simulink model "PhaseII_opalrt_NoProtection"  (Simulink 8.8)
settings: Solver=ode3  StartTime=0.0  StopTime=inf  FixedStep=Ts  RelTol=1e-5  EnableMultiTasking=on
PostLoadFcn:
  | %BESS ctrl
  | Kpf=0.005*3*12;
  | Kif=5*6;
  | 
  | Kpf1=0.005*3*12;
  | Kif1=5*6;
  | Kp_v=0.016*15*35;
  | Ki_v=12*25;
  | 
  | Kp_v1=0.016*15*35;
  | Ki_v1=12*25;
  | 
  | Vabc_B=12.47e3;
  | Vdc_ref=Vabc_B*2;
  | Kpwm=sqrt(2)*Vabc_B/Vdc_ref;
  | ZB=Vabc_B^2/1e6;
  | R=0.005*ZB;
  | Ibasefull=673/2*sqrt(2);
  | 
  | 
  | Ts_Control=1e-4;
  | ts=0.05;
  | delay=0.2;
  | offset=10e3;
  | t_plan=60;
  | t_monitor=.2;
  | t_mon=t_monitor;
  | scalingfactor=1;
  | x=0.5;
  | n=6;
  | %t_plan=1/15;
  | %t_monitor=10/900;
  | %t_mon=10/900;
  | 
  | %t_plan=1/5;
  | %t_monitor=10/300;
  | %t_mon=10/300;
  | %scalingfactor=1/300;
  | 
  | f0=60;
  | 
  | Pabc_B=1e6;
  | Iabc_B=Pabc_B*sqrt(2/3)/Vabc_B;  % pk value
  | Imax_1=2.5;
  | Ptrans_B=Pabc_B*200;
  | 
  | Vdc_ref=Vabc_B*2;
  | 
  | ZB=Vabc_B^2/Pabc_B;
  | L=0.1*ZB/2/pi/60;
  | R=0.1*ZB;
  | C=1/(4*pi^2*(2e3)^2*L);
  | 
  | LL=0.005*ZB/2/pi/60;
  | RR=0.005*ZB;
  | 
  | RC=0.02;
  | 
  | %%% Initial SOC %%%%
  | SOC_ini_BESS1=0.5;
  | ... (+223 lines)
InitFcn:
  | %BESS ctrl
  | Kpf=0.005*3*12;
  | Kif=5*6;
  | 
  | Kpf1=0.005*3*12;
  | Kif1=5*6;
  | Kp_v=0.016*15*35;
  | Ki_v=12*25;
  | 
  | Kp_v1=0.016*15*35;
  | Ki_v1=12*25;
  | 
  | Vabc_B=12.47e3;
  | Vdc_ref=Vabc_B*2;
  | Kpwm=sqrt(2)*Vabc_B/Vdc_ref;
  | ZB=Vabc_B^2/1e6;
  | R=0.005*ZB;
  | Ibasefull=673/2*sqrt(2);
  | 
  | 
  | Ts_Control=1e-4;
  | ts=0.05;
  | delay=0.2;
  | offset=10e3;
  | t_plan=60;
  | t_monitor=.2;
  | t_mon=t_monitor;
  | scalingfactor=1;
  | x=0.5;
  | n=6;
  | %t_plan=1/15;
  | %t_monitor=10/900;
  | %t_mon=10/900;
  | 
  | %t_plan=1/5;
  | %t_monitor=10/300;
  | %t_mon=10/300;
  | %scalingfactor=1/300;
  | 
  | f0=60;
  | 
  | Pabc_B=1e6;
  | Iabc_B=Pabc_B*sqrt(2/3)/Vabc_B;  % pk value
  | Imax_1=2.5;
  | Ptrans_B=Pabc_B*200;
  | 
  | Vdc_ref=Vabc_B*2;
  | 
  | ZB=Vabc_B^2/Pabc_B;
  | L=0.1*ZB/2/pi/60;
  | R=0.1*ZB;
  | C=1/(4*pi^2*(2e3)^2*L);
  | 
  | LL=0.005*ZB/2/pi/60;
  | RR=0.005*ZB;
  | 
  | RC=0.02;
  | 
  | %%% Initial SOC %%%%
  | SOC_ini_BESS1=0.5;
  | ... (+223 lines)
undefined symbols (not defined in the file): D1, Delta, DiscIntNeverNeededParam, Left, PG2ref, type, V
libraries: powerlib x220, powerlib_meascontrol x82, dspstat3 x54, dsparch4 x43, dspswit3 x24, simulink x19, simulink_extras x12, powerlib_extras x11, ssn_lib x7, artemis x6, rtlab x5, rtio_generic_dnp3 x5
(part 5 of 9)

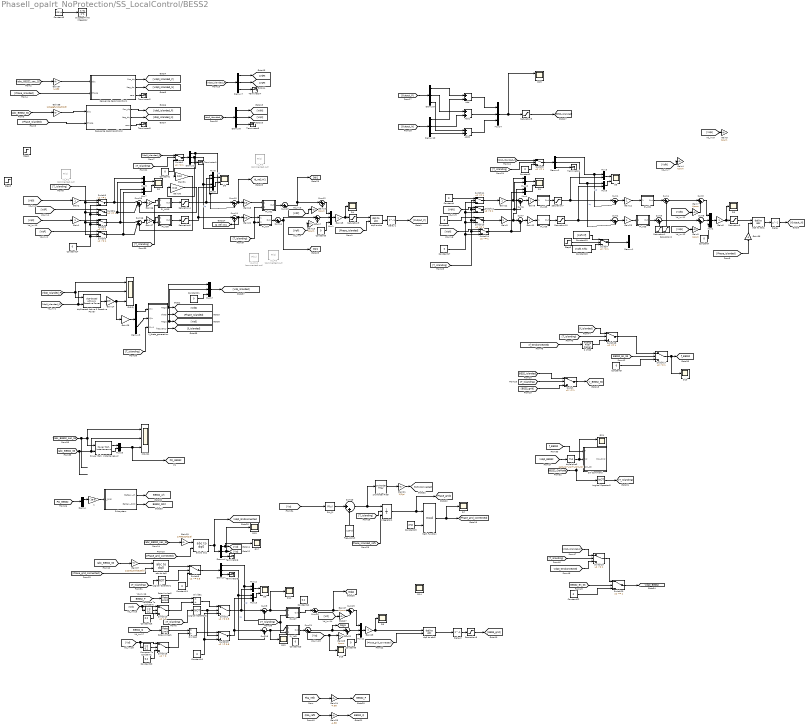
== system PhaseII_opalrt_NoProtection/SS_LocalControl/BESS2 ==
  "     1" : Gain  Gain=-1e-6
  2 kHz5 : dsparch4/Analog Filter Design  method=Butterworth  filttype=Lowpass  N=2  Wlo=2*pi*1  Whi=80  Rp=2  Rs=40
  2nd-Order Filter : powerlib_extras/Control  Blocks/2nd-Order Filter  FilterType=Lowpass  Fo=25  Zeta=0.707  Initialize=on  Vac_Init=[0 0 60]  Vdc_Init=377  PlotResponse=off  param1=[1 1000 0.5]
  Add : Sum
  Add1 : Sum
  Add2 : Sum
  Compare To Constant : simulink/Logic and Bit Operations/Compare To Constant  relop=>=  const=0.2  OutDataTypeStr=boolean
  Compare To Constant1 : simulink/Logic and Bit Operations/Compare To Constant  relop=>=  const=0.2  OutDataTypeStr=boolean
  Constant{1..2,4..11,13..14,17,21..22} (15 alike) : Constant  Value=0  SampleTime=-1
  Constant12 : Constant  Value=0.1  SampleTime=-1
  Constant15 : Constant  Value=2*pi
  Constant16 : Constant  Value=0.2  SampleTime=-1
  Constant18 : Constant  Value=[Kpf1 Kif1]  SampleTime=-1
  Constant19 : Constant  Value=[Kpf Kif]  SampleTime=-1
  Constant20 : Constant  Value=0.2  SampleTime=-1
  Constant3 : Constant  Value=120*pi
  D{1..2,5..6,9,15} (6 alike) : Scope  NumInputPorts=2
  D{3..4,7..8,10..14,16..17} (11 alike) : Scope
  D21 : Scope  NumInputPorts=3
  Delay : Delay  DelayLength=1  InitialCondition=0
  Delay1 : Delay  DelayLength=1  InitialCondition=0
  Delay2 : Delay  DelayLength=1  InitialCondition=0
  Demux : Demux  Outputs=2
  Demux1 : Demux  Outputs=2
  Demux{2,4..10} (8 alike) : Demux  Outputs=3
  Demux3 : Demux  Outputs=2
  Discrete-Time Integrator : DiscreteIntegrator  SampleTime=-1  ICPrevOutput=DiscIntNeverNeededParam  ICPrevScaledInput=DiscIntNeverNeededParam
  Divide1 : Product  Inputs=*/
  Divide2 : Product  Inputs=*/
  Freq_Const : Constant  Value=120*pi
  Gain{1..3,6,8,11..12,15,22..23,29} (11 alike) : Gain
  Gain{4..5,7,9..10,13,27..28} (8 alike) : Gain  Gain=Kpwm
  Gain14 : Gain  Gain=2/3
  Gain{16..18,20} (4 alike) : Gain  Gain=0.5
  Gain19 : Gain  Gain=1/480/sqrt(2/3)
  Gain21 : Gain  Gain=1/2/pi
  Gain24 : Gain  Gain=-4.38
  Gain25 : Gain  Gain=-4.38
  Gain26 : Gain  Gain=0.228
  Gain30 : Gain  Gain=0.12
  Gain31 : Gain  Gain=0.12
  Gain36 : Gain  Gain=-1
  Gain37 : Gain  Gain=1/sqrt(2/3)/Ibasefull
  Gain38 : Gain  Gain=1/Ibasefull/sqrt(2/3)
  Gain57 : Gain  Gain=1/480
  ID&IQ : Scope  NumInputPorts=3
  ID&IQ1 : Scope  NumInputPorts=3
  Integrator1 : Integrator  ExternalReset=falling  InitialConditionSource=external  LimitOutput=on
  Logical Operator1 : Logic  Operator=NOT  Inputs=1  AllPortsSameDT=off  OutDataTypeStr=boolean
  Logical Operator2 : Logic  Operator=NOT  Inputs=1  AllPortsSameDT=off  OutDataTypeStr=boolean
  Logical Operator3 : Logic  Operator=NOT  AllPortsSameDT=off  OutDataTypeStr=boolean
  Math Function : Math  Operator=mod  SaturateOnIntegerOverflow=on
  Mux{1..2,11,14,17} (5 alike) : Mux  Inputs=3
  Mux{3..10,12..13,16} (11 alike) : Mux  Inputs=2
  PI_Vd1 : Subsystem
  PI_Vd10 : Subsystem
  PI_Vd2 : Subsystem
  PI_Vd3 : Subsystem
  PI_Vd4 : Subsystem
  PI_Vd5 : Subsystem
  PI_Vd6 : Subsystem
  PI_Vd7 : Subsystem
  PI_Vd8 : Subsystem
  PI_Vd9 : Subsystem
  PLL_PI : simulink/Continuous/PID Controller  Controller=PI  TimeDomain=Continuous-time  SampleTime=-1  IntegratorMethod=Forward Euler  FilterMethod=Forward Euler  Form=Parallel  UseFilter=on  ControllerParametersSource=internal  P=53*100  I=900*100  D=0  N=100  InitialConditionSource=internal  InitialConditionForIntegrator=0  InitialConditionForFilter=0  ExternalReset=none  ZeroCross=off  LimitOutput=on  UpperSaturationLimit=20  LowerSaturationLimit=-20  LinearizeAsGain=off  AntiWindupMode=clamping  Kb=1  TrackingMode=off  Kt=1  PParamMin=[]  PParamMax=[]  IParamMin=[]  IParamMax=[]  DParamMin=[]  DParamMax=[]  NParamMin=[]  NParamMax=[]  KbParamMin=[]  KbParamMax=[]  KtParamMin=[]  KtParamMax=[]  POutMin=[]  POutMax=[]  IOutMin=[]  IOutMax=[]  DOutMin=[]  DOutMax=[]  NOutMin=[]  NOutMax=[]  KbOutMin=[]  KbOutMax=[]  KtOutMin=[]  KtOutMax=[]  IntegratorOutMin=[]  IntegratorOutMax=[]  FilterOutMin=[]  FilterOutMax=[]  SumOutMin=[]  SumOutMax=[]  SumI1OutMin=[]  SumI1OutMax=[]  SumI2OutMin=[]  SumI2OutMax=[]  SumI3OutMin=[]  SumI3OutMax=[]  SumDOutMin=[]  SumDOutMax=[]  SaturationOutMin=[]  SaturationOutMax=[]  IntegratorContinuousStateAttributes=''  IntegratorStateMustResolveToSignalObject=off  IntegratorRTWStateStorageClass=Auto  FilterContinuousStateAttributes=''  FilterStateMustResolveToSignalObject=off  FilterRTWStateStorageClass=Auto  DifferentiatorICPrevScaledInput=0  DifferentiatorOutMin=[]  DifferentiatorOutMax=[]
  "Power (3ph, Instantaneous)" : powerlib_meascontrol/Measurements/Power (3ph, Instantaneous)
  Rate Limiter1 : RateLimiter  RisingSlewLimit=10  FallingSlewLimit=-10  SampleTimeMode=inherited
  Rate Limiter2 : RateLimiter  RisingSlewLimit=10  FallingSlewLimit=-10  SampleTimeMode=inherited
  SW Command : Subsystem
  Saturation1 : Saturate  UpperLimit=0.95  LowerLimit=-0.95
  Saturation10 : Saturate  UpperLimit=0.15  LowerLimit=-0.15  ZeroCross=off
  Saturation2 : Saturate  UpperLimit=0.95  LowerLimit=-0.95
  Saturation3 : Saturate  UpperLimit=1  LowerLimit=-1
  Saturation4 : Saturate  UpperLimit=2.2  LowerLimit=-2.2  ZeroCross=off
  Saturation5 : Saturate  UpperLimit=1.1  LowerLimit=-1.1  ZeroCross=off
  Saturation6 : Saturate  UpperLimit=2.2  LowerLimit=-2.2  ZeroCross=off
  Saturation7 : Saturate  UpperLimit=0.15  LowerLimit=-0.15  ZeroCross=off
  Saturation8 : Saturate  UpperLimit=1  LowerLimit=-1  ZeroCross=off
  Saturation9 : Saturate  UpperLimit=1  LowerLimit=-1  ZeroCross=off
  Sequence decomposition1 : Subsystem
  Sequence decomposition2 : Subsystem
  Step1 : Step  Time=0.5  SampleTime=0  ZeroCross=off
  Step3 : Step  Time=0.5  SampleTime=0  ZeroCross=off
  Step6 : Step  Time=0.35  SampleTime=0
  Subsystem : Subsystem  mask{AH=100}
      mask prompts: AH "Capacity[Ah]"
      mask Display: image(imread(fullfile(matlabroot,'toolbox/physmod/powersys/DR/DRdemo/Battery.jpg')))
  Sum{1..2,6..7,9..11,18} (8 alike) : Sum  Inputs=|-+
  Sum{3,5,8,12,14,17,19,21..23} (10 alike) : Sum  Inputs=|++
  Sum13 : Sum  Inputs=|+-
  Sum15 : Sum  Inputs=|-++
  Sum16 : Sum  Inputs=|-+-
  Sum20 : Sum  Inputs=|+-
  Sum4 : Sum  Inputs=|+-
  Switch{,7,14,17..20} (7 alike) : Switch  Threshold=1
  Switch{1,3..6,9,11..13} (9 alike) : Switch  Threshold=1  ZeroCross=off
  Switch10 : Switch  Criteria=u2 > Threshold
  Switch15 : Switch  Threshold=0.5  ZeroCross=off
  Switch16 : Switch  Criteria=u2 > Threshold
  Switch2 : Switch  Threshold=0.5  ZeroCross=off
  Switch8 : Switch  Threshold=0.5  ZeroCross=off
  Terminator{1..8} (8 alike) : Terminator
  V_theta_generation : Subsystem
  Vd_PI10 : simulink/Continuous/PID Controller  Commented=on  Controller=PI  TimeDomain=Continuous-time  SampleTime=-1  IntegratorMethod=Trapezoidal  FilterMethod=Forward Euler  Form=Parallel  UseFilter=on  ControllerParametersSource=internal  P=Kpf1*5  I=Kif1*5  D=0  N=100  InitialConditionSource=internal  InitialConditionForIntegrator=0  InitialConditionForFilter=0  ExternalReset=none  LimitOutput=on  UpperSaturationLimit=1.2  LowerSaturationLimit=-1.2  LinearizeAsGain=off  AntiWindupMode=back-calculation  Kb=20  TrackingMode=off  Kt=1  PParamMin=[]  PParamMax=[]  IParamMin=[]  IParamMax=[]  DParamMin=[]  DParamMax=[]  NParamMin=[]  NParamMax=[]  KbParamMin=[]  KbParamMax=[]  KtParamMin=[]  KtParamMax=[]  POutMin=[]  POutMax=[]  IOutMin=[]  IOutMax=[]  DOutMin=[]  DOutMax=[]  NOutMin=[]  NOutMax=[]  KbOutMin=[]  KbOutMax=[]  KtOutMin=[]  KtOutMax=[]  IntegratorOutMin=[]  IntegratorOutMax=[]  FilterOutMin=[]  FilterOutMax=[]  SumOutMin=[]  SumOutMax=[]  SumI1OutMin=[]  SumI1OutMax=[]  SumI2OutMin=[]  SumI2OutMax=[]  SumI3OutMin=[]  SumI3OutMax=[]  SumDOutMin=[]  SumDOutMax=[]  SaturationOutMin=[]  SaturationOutMax=[]  IntegratorContinuousStateAttributes=''  IntegratorStateMustResolveToSignalObject=off  IntegratorRTWStateStorageClass=Auto  FilterContinuousStateAttributes=''  FilterStateMustResolveToSignalObject=off  FilterRTWStateStorageClass=Auto  DifferentiatorICPrevScaledInput=0  DifferentiatorOutMin=[]  DifferentiatorOutMax=[]
  Vd_PI2 : simulink/Continuous/PID Controller  Commented=on  Controller=PI  TimeDomain=Discrete-time  SampleTime=-1  IntegratorMethod=Forward Euler  FilterMethod=Forward Euler  Form=Parallel  UseFilter=on  ControllerParametersSource=internal  P=0.016*20  I=5*20  D=0  N=100  InitialConditionSource=internal  InitialConditionForIntegrator=0  InitialConditionForFilter=0  ExternalReset=none  LimitOutput=on  UpperSaturationLimit=0.5  LowerSaturationLimit=-0.5  LinearizeAsGain=off  AntiWindupMode=back-calculation  Kb=20  TrackingMode=off  Kt=1  PParamMin=[]  PParamMax=[]  IParamMin=[]  IParamMax=[]  DParamMin=[]  DParamMax=[]  NParamMin=[]  NParamMax=[]  KbParamMin=[]  KbParamMax=[]  KtParamMin=[]  KtParamMax=[]  POutMin=[]  POutMax=[]  IOutMin=[]  IOutMax=[]  DOutMin=[]  DOutMax=[]  NOutMin=[]  NOutMax=[]  KbOutMin=[]  KbOutMax=[]  KtOutMin=[]  KtOutMax=[]  IntegratorOutMin=[]  IntegratorOutMax=[]  FilterOutMin=[]  FilterOutMax=[]  SumOutMin=[]  SumOutMax=[]  SumI1OutMin=[]  SumI1OutMax=[]  SumI2OutMin=[]  SumI2OutMax=[]  SumI3OutMin=[]  SumI3OutMax=[]  SumDOutMin=[]  SumDOutMax=[]  SaturationOutMin=[]  SaturationOutMax=[]  IntegratorContinuousStateAttributes=''  IntegratorStateMustResolveToSignalObject=off  IntegratorRTWStateStorageClass=Auto  FilterContinuousStateAttributes=''  FilterStateMustResolveToSignalObject=off  FilterRTWStateStorageClass=Auto  DifferentiatorICPrevScaledInput=0  DifferentiatorOutMin=[]  DifferentiatorOutMax=[]
  Vd_PI6 : simulink/Continuous/PID Controller  Commented=on  Controller=PI  TimeDomain=Continuous-time  SampleTime=-1  IntegratorMethod=Forward Euler  FilterMethod=Forward Euler  Form=Parallel  UseFilter=on  ControllerParametersSource=internal  P=0.016*10  I=5*10  D=0  N=100  InitialConditionSource=internal  InitialConditionForIntegrator=0  InitialConditionForFilter=0  ExternalReset=none  LimitOutput=on  UpperSaturationLimit=3  LowerSaturationLimit=-3  LinearizeAsGain=off  AntiWindupMode=back-calculation  Kb=50  TrackingMode=off  Kt=1  PParamMin=[]  PParamMax=[]  IParamMin=[]  IParamMax=[]  DParamMin=[]  DParamMax=[]  NParamMin=[]  NParamMax=[]  KbParamMin=[]  KbParamMax=[]  KtParamMin=[]  KtParamMax=[]  POutMin=[]  POutMax=[]  IOutMin=[]  IOutMax=[]  DOutMin=[]  DOutMax=[]  NOutMin=[]  NOutMax=[]  KbOutMin=[]  KbOutMax=[]  KtOutMin=[]  KtOutMax=[]  IntegratorOutMin=[]  IntegratorOutMax=[]  FilterOutMin=[]  FilterOutMax=[]  SumOutMin=[]  SumOutMax=[]  SumI1OutMin=[]  SumI1OutMax=[]  SumI2OutMin=[]  SumI2OutMax=[]  SumI3OutMin=[]  SumI3OutMax=[]  SumDOutMin=[]  SumDOutMax=[]  SaturationOutMin=[]  SaturationOutMax=[]  IntegratorContinuousStateAttributes=''  IntegratorStateMustResolveToSignalObject=off  IntegratorRTWStateStorageClass=Auto  FilterContinuousStateAttributes=''  FilterStateMustResolveToSignalObject=off  FilterRTWStateStorageClass=Auto  DifferentiatorICPrevScaledInput=0  DifferentiatorOutMin=[]  DifferentiatorOutMax=[]
  Vd_PI8 : simulink/Continuous/PID Controller  Commented=on  Controller=PI  TimeDomain=Continuous-time  SampleTime=-1  IntegratorMethod=Trapezoidal  FilterMethod=Forward Euler  Form=Parallel  UseFilter=on  ControllerParametersSource=internal  P=Kpf1*5  I=Kif1*5  D=0  N=100  InitialConditionSource=internal  InitialConditionForIntegrator=0  InitialConditionForFilter=0  ExternalReset=none  LimitOutput=on  UpperSaturationLimit=1.2  LowerSaturationLimit=-1.2  LinearizeAsGain=off  AntiWindupMode=back-calculation  Kb=20  TrackingMode=off  Kt=1  PParamMin=[]  PParamMax=[]  IParamMin=[]  IParamMax=[]  DParamMin=[]  DParamMax=[]  NParamMin=[]  NParamMax=[]  KbParamMin=[]  KbParamMax=[]  KtParamMin=[]  KtParamMax=[]  POutMin=[]  POutMax=[]  IOutMin=[]  IOutMax=[]  DOutMin=[]  DOutMax=[]  NOutMin=[]  NOutMax=[]  KbOutMin=[]  KbOutMax=[]  KtOutMin=[]  KtOutMax=[]  IntegratorOutMin=[]  IntegratorOutMax=[]  FilterOutMin=[]  FilterOutMax=[]  SumOutMin=[]  SumOutMax=[]  SumI1OutMin=[]  SumI1OutMax=[]  SumI2OutMin=[]  SumI2OutMax=[]  SumI3OutMin=[]  SumI3OutMax=[]  SumDOutMin=[]  SumDOutMax=[]  SaturationOutMin=[]  SaturationOutMax=[]  IntegratorContinuousStateAttributes=''  IntegratorStateMustResolveToSignalObject=off  IntegratorRTWStateStorageClass=Auto  FilterContinuousStateAttributes=''  FilterStateMustResolveToSignalObject=off  FilterRTWStateStorageClass=Auto  DifferentiatorICPrevScaledInput=0  DifferentiatorOutMin=[]  DifferentiatorOutMax=[]
  abc to dq0 : powerlib_meascontrol/Transformations/abc to dq0  Alignment=90 degrees behind phase A axis
  abc to dq1 : powerlib_meascontrol/Transformations/abc to dq0  Alignment=90 degrees behind phase A axis
  dq0 to abc : powerlib_meascontrol/Transformations/dq0 to abc  Alignment=90 degrees behind phase A axis
  dq0 to abc1 : powerlib_meascontrol/Transformations/dq0 to abc  Alignment=90 degrees behind phase A axis
  dq0 to abc2 : powerlib_meascontrol/Transformations/dq0 to abc  Alignment=90 degrees behind phase A axis
  dq0-based Active & Reactive Power : powerlib_extras/Measurements/dq0-based Active & Reactive Power
  dq2alpha3 : Fcn  Expr=sqrt(u(1)*u(1)+u(2)*u(2))
  tag scope: BESS2_Ah=global, BESS2_P=global, BESS2_Q=global, BESS2_SOC=global, Ddg1=global, Ddi1=global, Dqg1=global, Dqi1=global, Id_ref_ini1=global, Iq_ref_ini1=global, PQ_BESS2=global, Phase_grid2=global, V_BESS2_SS=global, Vdq0_BESS2=global, Vdq0_Gridconnected=global, f_BESS2=global
  wires:
  Mux9/1 -> D2/1
  Demux5/1 -> Gain31/1, Sum10/2, Mux6/1  "Id"
  Constant5/1 -> Mux1/3
  Sum14/1 -> Sum17/1, [Dqi1]
  PI_Vd1/1(Out) -> Sum13/1
  Gain17/1 -> PI_Vd8/1(Error)
  Gain16/1 -> PI_Vd10/1(Error)
  Sum15/1 -> Gain16/1
  Demux5/3 -> Terminator1/1
  [VqP] -> Gain13/1
  Mux8/1 -> D6/2
  Mux1/1 -> Gain15/1
  Sum12/1 -> Mux1/1
  [Vq0] -> Gain1/1
  Gain20/1 -> PI_Vd4/1(Error)
  Sum13/1 -> [Ddi1], Sum12/1
  PI_Vd4/1(Out) -> Sum14/1
  Gain15/1 -> Saturation9/1, D4/1
  [VdP] -> Gain10/1
  Sum16/1 -> Gain17/1
  Demux5/2 -> Gain30/1, Mux8/1, Sum11/2  "Iq"
  Mux7/1 -> D2/2
  Gain18/1 -> PI_Vd1/1(Error)
  Mux6/1 -> D6/1
  Sum10/1 -> [Id_ref_ini1], Gain18/1
  Sum11/1 -> [Iq_ref_ini1], Gain20/1
  [Vd0] -> Gain2/1
  Sum17/1 -> Mux1/2
  [Vabc_BESS2_sec_SS] -> Gain57/1
  [Iabc_BESS2_SS] -> Gain38/1
  Constant3/1 -> Discrete-Time Integrator/1
  [Phase_islanded] -> Sequence decomposition1/2(Phase)
  [Phase_islanded] -> Sequence decomposition2/2(Phase)
  Sequence decomposition1/1(Pos_dq) -> [Vdq0_islanded_P]
  Sequence decomposition1/2(Neg_dq) -> [Vdq0_islanded_N]
  Sequence decomposition1/3(zero) -> Terminator2/1
  Sequence decomposition2/1(Pos_dq) -> [Idq0_islanded_P]
  Sequence decomposition2/2(Neg_dq) -> [Idq0_islanded_N]
  Sequence decomposition2/3(zero) -> Terminator3/1
  Saturation9/1 -> dq0 to abc/1
  [Phase_islanded] -> dq0 to abc/2
  Constant7/1 -> Mux2/3
  Sum7/1 -> Gain11/1
  Mux3/1 -> D5/1
  Switch14/1 -> Sum7/2, Mux4/2
  Mux4/1 -> D1/2
  Sum1/1 -> Gain12/1
  Gain11/1 -> PI_Vd6/1(Error)
  Sum5/1 -> Sum8/1
  Mux10/1 -> D1/1
  Demux2/3 -> Terminator4/1
  Gain22/1 -> Mux10/1, Sum6/1
  Saturation1/1 -> Sum5/2
  Sum2/1 -> Gain23/1
  Gain12/1 -> PI_Vd2/1(Error)
  Sum6/1 -> Gain8/1
  PI_Vd3/1(Out) -> Sum5/1
  Sum4/1 -> Sum3/1
  Saturation2/1 -> Sum4/2
  Gain6/1 -> D3/1, Saturation3/1
  Switch12/1 -> Mux10/2, Sum6/2
  Gain3/1 -> Mux4/1, Sum7/1
  Mux5/1 -> D5/2
  [VqN] -> Gain5/1
  PI_Vd2/1(Out) -> Sum4/1
  [VdN] -> Gain4/1
  [Phase_islanded] -> Gain36/1
  Mux2/1 -> Gain6/1
  Saturation3/1 -> dq0 to abc1/1
  [Vdq0_islanded_P] -> Demux7/1
  Demux7/1 -> [VdP]
  Demux7/2 -> [VqP]
  Demux7/3 -> Terminator7/1
  Demux8/1 -> [VdN]
  Demux8/3 -> Terminator8/1
  Demux8/2 -> [VqN]
  [Vdq0_islanded_N] -> Demux8/1
  Gain36/1 -> dq0 to abc1/2
  [Output_P] -> Demux9/1
  [Output_N] -> Demux10/1
  Demux9/1 -> Add/1
  Demux10/1 -> Add/2
  Demux9/2 -> Add1/1
  Demux10/2 -> Add1/2
  Demux9/3 -> Add2/1
  Demux10/3 -> Add2/2
  Add1/1 -> Mux14/2
  Add/1 -> Mux14/1
  Add2/1 -> Mux14/3
  Mux14/1 -> D15/1, Saturation5/1
  Gain2/1 -> Switch3/1
  [VdP] -> Switch4/1
  Gain1/1 -> Switch5/1
  [VqP] -> Switch6/1
  Constant14/1 -> Switch6/3, Switch5/3, Switch4/3, Switch3/3
  Switch3/1 -> Mux9/1, Sum15/1
  Switch4/1 -> Mux9/2, Sum15/2
  Switch5/1 -> Mux7/1, Sum16/1
  Switch6/1 -> Mux7/2, Sum16/2
  PI_Vd10/1(Out) -> Saturation4/1
  Switch11/1 -> Gain22/1
  Constant4/1 -> Switch11/1
  [VqN] -> Switch14/1
  Switch13/1 -> Gain3/1
  Constant6/1 -> Switch13/1
  [VdN] -> Switch12/1
  Constant17/1 -> Switch14/3, Switch13/3, Switch12/3, Switch11/3
  [T_islanding] -> Switch14/2, Switch13/2, Switch12/2, Switch11/2
  Demux2/1 -> Sum1/2, Mux3/1  "Id"
  Demux2/2 -> Sum2/2, Mux5/1  "Iq"
  Gain38/1 -> Sequence decomposition2/1(abc)
  Gain57/1 -> Sequence decomposition1/1(abc)
  Gain23/1 -> PI_Vd3/1(Error)
  Sum3/1 -> Mux2/1
  Sum8/1 -> Mux2/2
  PI_Vd8/1(Out) -> Saturation6/1
  Step6/1 -> Switch7/2
  Constant18/1 -> Switch7/3
  Switch7/1 -> Demux1/1
  Constant19/1 -> Switch7/1
  [VdN] -> Gain7/1
  [VqN] -> Gain9/1
  Gain10/1 -> Sum12/2
  Gain13/1 -> Sum17/2
  Gain7/1 -> Sum3/2
  Gain9/1 -> Sum8/2
  Saturation5/1 -> [BESS_islanded]
  Gain8/1 -> PI_Vd5/1(Error)
  Delay1/1 -> [Output_P]
  dq0 to abc1/1 -> Delay/1
  Delay/1 -> [Output_N]
  dq0 to abc/1 -> Delay1/1
  Demux6/2 -> D13/1, [Vq]
  dq0 to abc2/1 -> Delay2/1
  Delay2/1 -> Saturation8/1
  Gain37/1 -> abc to dq0/1
  Demux4/3 -> Terminator5/1
  Sum9/1 -> PI_Vd7/1(Error), D11/1
  Switch8/1 -> Demux4/1
  Freq_Const/1 -> Sum23/2
  [Phase_grid_connected] -> abc to dq1/2
  [Phase_grid_connected] -> abc to dq0/2
  Demux6/3 -> Terminator6/1
  Sum18/1 -> PI_Vd9/1(Error), D12/1
  Constant8/1 -> Mux11/3
  Mux13/1 -> D9/2
  PI_Vd9/1(Out) -> Sum21/1
  Sum21/1 -> [Dqg1], Sum22/1
  Sum22/1 -> Mux11/2
  Mux11/1 -> Gain29/1
  [Vq] -> PLL_PI/1
  PI_Vd7/1(Out) -> Sum20/1
  PLL_PI/1 -> Sum23/1
  [Iabc_BESS2_SS] -> Gain37/1
  [Vd] -> Gain27/1
  abc to dq0/1 -> Switch8/1
  Switch2/1 -> Mux12/2, Sum9/1
  Mux12/1 -> D9/1
  Constant11/1 -> Switch8/3
  Demux4/1 -> Mux12/1, Sum9/2  "Id"
  Integrator1/1 -> [Phase_grid2], Math Function/1
  [Phase_grid_connected] -> dq0 to abc2/2
  Demux6/1 -> D17/1, [Vd]
  Demux4/2 -> Mux13/1, Sum18/2  "Iq"
  Sum20/1 -> [Ddg1], Sum19/1
  Gain29/1 -> dq0 to abc2/1, D8/1
  [Vq] -> D16/1, Gain28/1
  Sum19/1 -> Mux11/1
  Constant15/1 -> Math Function/2
  [Vabc_BESS2_sec_SS] -> Gain19/1
  Gain19/1 -> abc to dq1/1
  Math Function/1 -> D7/1, [Phase_grid_connected]
  Saturation8/1 -> [BESS_grid]
  Switch1/1 -> Demux5/1
  [Idq0_islanded_P] -> Switch1/1
  Constant1/1 -> Switch1/3
  Switch9/1 -> Demux2/1
  [Idq0_islanded_N] -> Switch9/1
  [T_islanding] -> Switch9/2
  Constant2/1 -> Switch9/3
  Saturation4/1 -> Sum10/1, Mux6/2
  Saturation6/1 -> Sum11/1, Mux8/2
  PI_Vd5/1(Out) -> Saturation7/1
  PI_Vd6/1(Out) -> Saturation10/1
  Saturation7/1 -> Sum1/1, Mux3/2
  Saturation10/1 -> Sum2/1, Mux5/2
  Constant16/1 -> Switch10/3
  Compare To Constant/1 -> Switch10/2
  [Vd] -> Compare To Constant/1, Switch10/1
  Switch10/1 -> Divide1/2
  [BESS2_P] -> Rate Limiter2/1
  Rate Limiter2/1 -> Divide1/1
  Divide1/1 -> Switch2/1
  [BESS2_Q] -> Rate Limiter1/1
  Divide2/1 -> Switch15/1
  Switch15/1 -> Sum18/1, Mux13/2
  Rate Limiter1/1 -> Divide2/1
  Compare To Constant1/1 -> Switch16/2
  [Vd] -> Compare To Constant1/1, Switch16/1
  Constant20/1 -> Switch16/3
  Switch16/1 -> Divide2/2
  Constant10/1 -> Switch15/3, Switch2/3
  [T_islanding] -> Switch3/2, Switch4/2, Switch5/2, Switch6/2
  [T_islanding] -> Switch1/2
  Gain27/1 -> Sum19/2
  Gain28/1 -> Sum22/2
  Demux3/1 -> V_theta_generation/1(Pin)
  Gain14/1 -> Gain26/1, ID&IQ/3
  [Vdq0_islanded_P] -> ID&IQ/1, dq0-based Active & Reactive Power/1
  V_theta_generation/3(Magq) -> Mux17/2, [Vq0]
  dq0-based Active & Reactive Power/1 -> Gain14/1
  V_theta_generation/2(theta) -> [Phase_islanded]
  [Idq0_islanded_P] -> ID&IQ/2, dq0-based Active & Reactive Power/2
  V_theta_generation/1(Magd) -> Mux17/1, [Vd0]
  Demux3/2 -> V_theta_generation/2(Qin)
  [T_islanding] -> Integrator1/2
  [Phase_islanded_ref1] -> Integrator1/3
  [T_islanding] -> Logical Operator1/1
  Logical Operator1/1 -> Switch8/2
  [T_islanding] -> Logical Operator2/1
  Logical Operator2/1 -> Switch15/2, Switch2/2
  [f_BESS2] -> SW Command/1(f)
  [Vdq0_BESS2] -> dq2alpha3/1
  dq2alpha3/1 -> D21/1, SW Command/2(Vd)
  [BESS2_OpMode] -> SW Command/3(SW_Ctr), Logical Operator3/1
  Sum23/1 -> 2nd-Order Filter/1, Integrator1/1
  Gain21/1 -> [f_Gridconnected]
  abc to dq1/1 -> [Vdq0_Gridconnected], Demux6/1
  [Vabc_BESS2_sec_SS] -> "Power (3ph, Instantaneous)"/1, ID&IQ1/1
  [Iabc_BESS2_SS] -> "Power (3ph, Instantaneous)"/2, ID&IQ1/2
  Mux16/1 -> [PQ_BESS2], ID&IQ1/3
  "     1"/1 -> Subsystem/1(I_RMS)
  Subsystem/2(Battery_SOC) -> [BESS2_SOC]
  Subsystem/1(Battery_Ah) -> [BESS2_Ah]
  Demux/1 -> "     1"/1
  [PQ_BESS2] -> Demux/1
  [T_islanding] -> PI_Vd8/2(T_islanding), PI_Vd10/2(T_islanding)
  [T_islanding] -> PI_Vd1/2(T_islanding), PI_Vd4/2(T_islanding)
  [T_islanding] -> PI_Vd7/2(T_islanding), PI_Vd9/2(T_islanding)
  Logical Operator3/1 -> [T_islanding]
  "Power (3ph, Instantaneous)"/1 -> Mux16/1
  "Power (3ph, Instantaneous)"/2 -> Mux16/2
  [T_islanding] -> V_theta_generation/3(Pin1)
  2nd-Order Filter/1 -> Gain21/1
  [T_islanding] -> Switch/2
  [BESS_islanded] -> Switch/1
  [BESS_grid] -> Switch/3
  Switch17/1 -> [f_BESS2], D10/1
  [BESS2_En_SS] -> Switch17/2
  Constant9/1 -> Switch17/3
  [T_islanding] -> Switch18/2
  [f_islanded] -> Switch18/1
  [f_Gridconnected] -> 2 kHz5/1
  [T_islanding] -> Switch19/2
  [Vdq0_islanded_P] -> Switch19/1
  [Vdq0_Gridconnected] -> Switch19/3
  V_theta_generation/4(frequency) -> [f_islanded]
  Mux17/1 -> [Vdq_islanded]
  Constant21/1 -> Mux17/3
  [Pba_ref2] -> Gain24/1
  [Qba_ref2] -> Gain25/1
  Switch18/1 -> Switch17/1
  [BESS2_En_SS] -> Switch20/2
  Constant22/1 -> Switch20/3
  Switch20/1 -> [Vdq0_BESS2]
  Switch19/1 -> Switch20/1
  Switch/1 -> [V_BESS2_SS]
  Gain24/1 -> [BESS2_P]
  Gain25/1 -> [BESS2_Q]
  Gain26/1 -> Demux3/1
  Gain30/1 -> Sum15/3
  Gain31/1 -> Sum16/3
  2 kHz5/1 -> Switch18/3

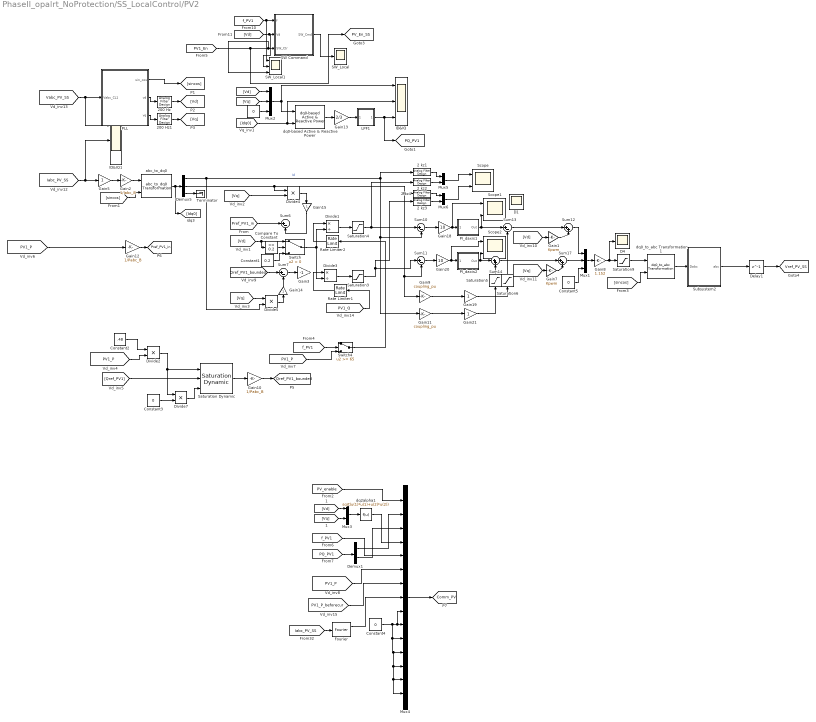
== system PhaseII_opalrt_NoProtection/SS_LocalControl/PV2 ==
  " " : Constant  Value=0
  2 kz{1..4} (4 alike) : dsparch4/Analog Filter Design  method=Butterworth  filttype=Lowpass  N=2  Wlo=2*pi*500  Whi=80  Rp=2  Rs=40
  200 Hz : dsparch4/Analog Filter Design  method=Butterworth  filttype=Lowpass  N=2  Wlo=2*pi*200  Whi=80  Rp=2  Rs=40
  200 Hz1 : dsparch4/Analog Filter Design  method=Butterworth  filttype=Lowpass  N=2  Wlo=2*pi*200  Whi=80  Rp=2  Rs=40
  Compare To Constant : simulink/Logic and Bit Operations/Compare To Constant  relop=>=  const=0.2  OutDataTypeStr=boolean
  Constant1 : Constant  Value=0.2  SampleTime=-1
  Constant2 : Constant  Value=.48
  Constant3 : Constant  Value=0
  Constant4 : Constant  Value=0
  Constant5 : Constant  Value=0  SampleTime=-1
  D1 : Scope
  D4 : Scope
  Delay1 : Delay  DelayLength=1  InitialCondition=0
  Demux1 : Demux  Outputs=2
  Demux5 : Demux  Outputs=3
  Divide1 : Product  Inputs=*/
  Divide{2,4..5,7} (4 alike) : Product  Inputs=**
  Divide3 : Product  Inputs=*/
  Fourier : powerlib_meascontrol/Measurements/Fourier  Freq=60  n=1  InInit=[0, 0]  Ts=0
  Gain1 : Gain  Gain=Kpwm
  Gain10 : Gain  Gain=1/Pabc_B
  Gain11 : Gain  Gain=coupling_pu
  Gain12 : Gain  Gain=1/Pabc_B
  Gain13 : Gain  Gain=2/3
  Gain{5,14..15,19,21} (5 alike) : Gain
  Gain18 : Gain  Gain=10
  Gain2 : Gain  Gain=1/Iabc_B
  Gain20 : Gain  Gain=10
  Gain3 : Gain  Gain=-1
  Gain7 : Gain  Gain=Kpwm
  Gain8 : Gain  Gain=1.152
  Gain9 : Gain  Gain=coupling_pu
  ID&IQ : Scope  NumInputPorts=3
  ID&IQ1 : Scope  NumInputPorts=3
  LPF1 : Subsystem
  Mux1 : Mux  Inputs=3
  Mux2 : Mux  Inputs=3
  Mux3 : Mux  Inputs=2
  Mux4 : Mux  Inputs=15
  Mux5 : Mux  Inputs=2
  Mux6 : Mux  Inputs=2
  PI_daxis1 : Subsystem
  PI_daxis2 : Subsystem
  "PLL " : Subsystem
  Rate Limiter1 : RateLimiter  RisingSlewLimit=0.2*100  FallingSlewLimit=-0.2*100  SampleTimeMode=inherited
  Rate Limiter2 : RateLimiter  RisingSlewLimit=100  FallingSlewLimit=-100  SampleTimeMode=inherited
  SW Command : Subsystem
  SW_Local : Scope
  SW_Local1 : Scope  NumInputPorts=3
  Saturation Dynamic : simulink/Discontinuities/Saturation Dynamic  OutMin=[]  OutMax=[]  OutDataTypeStr=Inherit: Same as second input  OutDataType=fixdt(1, 16)  OutScaling=2^-10  DoSatur=off
  Saturation3 : Saturate  UpperLimit=Imax_1  LowerLimit=-Imax_1
  Saturation4 : Saturate  UpperLimit=Imax_1  LowerLimit=-Imax_1
  Saturation5 : Saturate  UpperLimit=0.95  LowerLimit=-0.95
  Saturation6 : Saturate  UpperLimit=0.95  LowerLimit=-0.95
  Saturation9 : Saturate  UpperLimit=10  LowerLimit=-10
  Scope : Scope  NumInputPorts=2
  Scope1 : Scope  NumInputPorts=2
  Scope2 : Scope  NumInputPorts=2
  Subsystem2 : Subsystem
  Sum{6..7,10..11,13} (5 alike) : Sum  Inputs=|+-
  Sum12 : Sum  Inputs=|++
  Sum14 : Sum  Inputs=|++
  Sum17 : Sum  Inputs=|++
  Switch : Switch  Criteria=u2 > Threshold
  Switch4 : Switch  Threshold=65  ZeroCross=off
  Terminator : Terminator
  abc_to_dq0 : powerlib_extras/Measurements/abc_to_dq0 Transformation
  dq0-based Active & Reactive Power : powerlib_extras/Measurements/dq0-based Active & Reactive Power
  dq0_to_abc Transformation1 : powerlib_extras/Measurements/dq0_to_abc Transformation
  dq2alpha1 : Fcn  Expr=sqrt(u(1)*u(1)+u(2)*u(2))
  tag scope: Comm_PV=global, PQ_PV1=global, PV_En_SS=global, Pref_PV1_in=global, Qref_PV1_bounded=global, Vref_PV_SS=global
  wires:
  abc_to_dq0/1 -> Demux5/1, [Idq0]
  "PLL "/3(vq) -> 200 Hz1/1
  "PLL "/2(vd) -> 200 Hz/1
  "PLL "/1(sin_cos) -> [sincos]
  Divide5/1 -> Gain14/1
  [sincos] -> abc_to_dq0/2
  Gain15/1 -> Sum6/2
  Gain14/1 -> Sum7/2
  Divide4/1 -> Gain15/1
  [Vq] -> Divide4/2
  Sum7/1 -> Gain3/1
  [Qref_PV1_bounded] -> Sum7/1
  dq0-based Active & Reactive Power/1 -> Gain13/1
  Mux2/1 -> ID&IQ/1, dq0-based Active & Reactive Power/1
  " "/1 -> Mux2/3
  [Vq] -> Mux2/2
  [Vd] -> Mux2/1
  Demux5/3 -> Terminator/1
  Gain2/1 -> abc_to_dq0/1
  [Vd] -> SW_Local1/2, SW Command/2(Vd)
  [PV1_En] -> [PV_En_SS], SW_Local1/3, SW Command/3(SW_Ctr)
  Gain5/1 -> Gain2/1
  200 Hz/1 -> [Vd]
  200 Hz1/1 -> [Vq]
  SW Command/1(SW_Cmd) -> SW_Local/1
  [Idq0] -> ID&IQ/2, dq0-based Active & Reactive Power/2
  Gain13/1 -> LPF1/1(In1)
  LPF1/1(Out1) -> ID&IQ/3, [PQ_PV1]
  [PV1_P] -> Divide2/2
  Constant2/1 -> Divide2/1
  [Qref_PV1] -> Saturation Dynamic/2
  Divide2/1 -> Saturation Dynamic/1, Divide7/1
  Constant3/1 -> Divide7/2
  Divide7/1 -> Saturation Dynamic/3
  Sum12/1 -> Mux1/1
  PI_daxis1/1(Out) -> Sum13/1, Scope1/2
  Sum10/1 -> Gain18/1
  Mux1/1 -> Gain8/1
  Sum11/1 -> Gain20/1
  Gain20/1 -> Scope2/1, PI_daxis2/1(Error)
  PI_daxis2/1(Out) -> Scope2/2, Sum14/1
  Gain19/1 -> Saturation6/1
  Gain21/1 -> Saturation5/1
  Gain9/1 -> Gain19/1
  Gain11/1 -> Gain21/1
  [sincos] -> dq0_to_abc Transformation1/2
  [Vd] -> Gain1/1
  Sum17/1 -> Mux1/2
  [Vq] -> Gain7/1
  Constant5/1 -> Mux1/3
  Gain8/1 -> Saturation9/1, D4/1
  Saturation9/1 -> dq0_to_abc Transformation1/1
  dq0_to_abc Transformation1/1 -> Subsystem2/1(Dabc)
  Saturation5/1 -> Sum14/2
  Saturation6/1 -> Sum13/2
  Sum13/1 -> Sum12/1
  Sum14/1 -> Sum17/1
  Demux5/2 -> Divide4/1, 2 kz4/1, Sum11/2, Gain9/1
  Demux5/1 -> Divide5/2, 2 kz1/1, Sum10/2, Gain11/1  "Id"
  [Vd] -> Compare To Constant/1, Switch/1
  Compare To Constant/1 -> Switch/2
  Constant1/1 -> Switch/3
  [Vq] -> Divide5/1
  Switch/1 -> Divide3/2, Divide1/2
  Saturation Dynamic/1 -> Gain10/1
  [Pref_PV1_in] -> Sum6/1
  Divide1/1 -> Saturation4/1
  Divide3/1 -> Saturation3/1
  Gain12/1 -> [Pref_PV1_in]
  Gain10/1 -> [Qref_PV1_bounded]
  Subsystem2/1(abc) -> Delay1/1
  [f_PV1] -> SW_Local1/1, SW Command/1(f)
  Gain1/1 -> Sum12/2
  Gain7/1 -> Sum17/2
  Mux5/1 -> Scope/1
  Mux6/1 -> Scope/2
  2 kz1/1 -> Mux5/1
  2 kz2/1 -> Mux5/2
  2 kz4/1 -> Mux6/1
  2 kz3/1 -> Mux6/2
  [PV1_P] -> Gain12/1
  [Vq] -> Mux3/2
  [Vd] -> Mux3/1
  Mux3/1 -> dq2alpha1/1
  [PQ_PV1] -> Demux1/1
  [PV1_P] -> Mux4/6
  Constant4/1 -> Mux4/11, Mux4/15, Mux4/14, Mux4/13, Mux4/12, Mux4/10, Mux4/9
  Mux4/1 -> [Comm_PV]
  [Iabc_PV_SS] -> ID&IQ1/2, Gain5/1
  [Vabc_PV_SS] -> ID&IQ1/1, "PLL "/1(Vabc_CL1)
  [PV_enable] -> Mux4/1
  Gain18/1 -> Scope1/1, PI_daxis1/1(Error)
  Saturation4/1 -> Sum10/1, 2 kz2/1
  Saturation3/1 -> Sum11/1, 2 kz3/1
  [PV1_P_beforecur] -> Mux4/7
  [PV1_Q] -> Rate Limiter1/1
  Rate Limiter1/1 -> Divide3/1
  Rate Limiter2/1 -> Divide1/1
  [Iabc_PV_SS] -> Fourier/1
  Fourier/1 -> Mux4/8
  Delay1/1 -> [Vref_PV_SS]
  Demux1/1 -> Mux4/2
  Demux1/2 -> Mux4/3
  dq2alpha1/1 -> Mux4/4
  [f_PV1] -> Mux4/5
  [PV1_P] -> Switch4/3
  [f_PV1] -> Switch4/2
  Switch4/1 -> Rate Limiter2/1

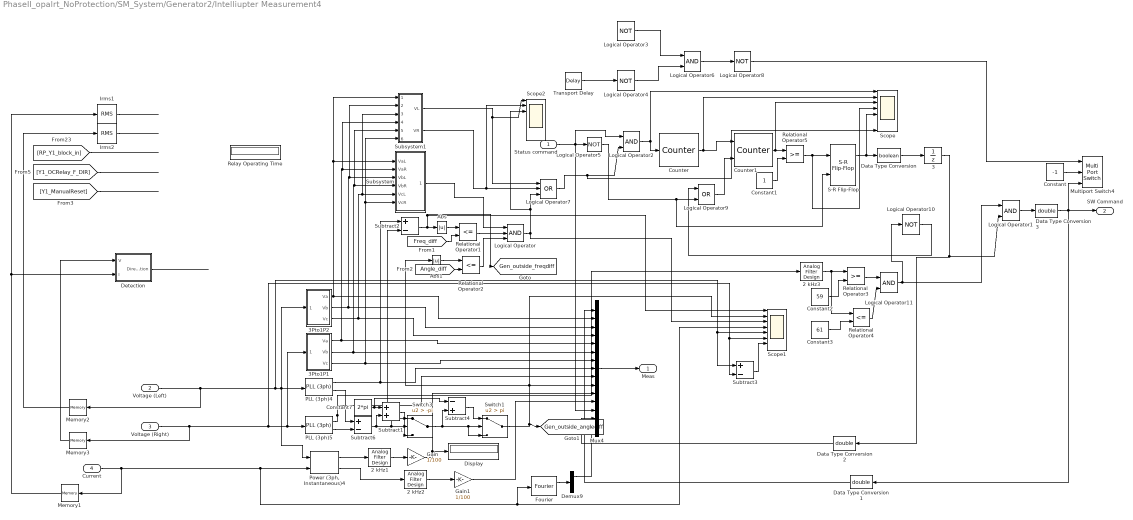
== system PhaseII_opalrt_NoProtection/SM_System/Generator2/Intelliupter Measurement4 ==
  Status command : Inport
  Voltage (Left) : Inport  Port=2
  Voltage (Right) : Inport  Port=3
  Current : Inport  Port=4
  "   3" : UnitDelay  SampleTime=Ts
  2 kHz1 : dsparch4/Analog Filter Design  method=Butterworth  filttype=Lowpass  N=2  Wlo=2*pi*0.1  Whi=80  Rp=2  Rs=40
  2 kHz2 : dsparch4/Analog Filter Design  method=Butterworth  filttype=Lowpass  N=2  Wlo=2*pi*0.1  Whi=80  Rp=2  Rs=40
  2 kHz3 : dsparch4/Analog Filter Design  method=Butterworth  filttype=Lowpass  N=2  Wlo=2*pi*0.1  Whi=80  Rp=2  Rs=40
  3Pto1P1 : Subsystem
  3Pto1P2 : Subsystem
  Abs : Abs
  Abs1 : Abs
  Constant : Constant  Value=-1
  Constant1 : Constant
  Constant2 : Constant  Value=59
  Constant3 : Constant  Value=61
  Constant7 : Constant  Value=2*pi
  Counter : dspswit3/Counter  Direction=Up  CountEvent=Non-zero sample  CounterSize=User defined  MaxCount=10000  InitialCount=0  Output=Hit  HitValue=2000  ResetInput=off  SamplesPerFrame=1  Ts=1  CntDtype=double  HitDtype=Logical
  Counter1 : dspswit3/Counter  Direction=Up  CountEvent=Non-zero sample  CounterSize=User defined  MaxCount=255  InitialCount=0  Output=Count  HitValue=50  ResetInput=on  SamplesPerFrame=1  Ts=1  CntDtype=double  HitDtype=Logical
  Data Type Conversion : DataTypeConversion  OutDataTypeStr=boolean
  Data Type Conversion1 : DataTypeConversion  OutDataTypeStr=double
  Data Type Conversion2 : DataTypeConversion  OutDataTypeStr=double
  Data Type Conversion3 : DataTypeConversion  OutDataTypeStr=double
  Demux9 : Demux  Outputs=3
  Detection : Subsystem
  Display : Display
  Fourier : powerlib_meascontrol/Measurements/Fourier  Freq=60  n=1  InInit=[0, 0]  Ts=0
  Gain : Gain  Gain=1/100
  Gain1 : Gain  Gain=1/100
  Irms1 : powerlib_meascontrol/Measurements/RMS  TrueRMS=on  Freq=60  RMSInit=0  Ts=0
  Irms2 : powerlib_meascontrol/Measurements/RMS  TrueRMS=on  Freq=60  RMSInit=0  Ts=0
  Logical Operator : Logic  Inputs=3  AllPortsSameDT=off  OutDataTypeStr=boolean
  Logical Operator1 : Logic
  Logical Operator{3..4,8,10} (4 alike) : Logic  Operator=NOT
  Logical Operator11 : Logic
  Logical Operator2 : Logic  AllPortsSameDT=off  OutDataTypeStr=boolean
  Logical Operator5 : Logic  Operator=NOT  AllPortsSameDT=off  OutDataTypeStr=boolean
  Logical Operator6 : Logic
  Logical Operator7 : Logic  Operator=OR  Inputs=3  AllPortsSameDT=off
  Logical Operator9 : Logic  Operator=OR  AllPortsSameDT=off  OutDataTypeStr=boolean
  Memory1 : Memory
  Memory2 : Memory
  Memory3 : Memory
  Multiport Switch4 : MultiPortSwitch  DataPortOrder=Zero-based contiguous  Inputs=2  DiagnosticForDefault=None
  Mux4 : Mux  Inputs=15
  PLL (3ph)4 : powerlib_meascontrol/PLL/PLL (3ph)  Fmin=45  Par_Init=[0, 60]  ParK=[180, 3200, 1]  TcD=1e-4  MaxRateChangeFreq=12  FilterCutOffFreq=25  Ts=0  AGC=on
  PLL (3ph)5 : powerlib_meascontrol/PLL/PLL (3ph)  Fmin=45  Par_Init=[0, 60]  ParK=[180, 3200, 1]  TcD=1e-4  MaxRateChangeFreq=12  FilterCutOffFreq=25  Ts=0  AGC=on
  "Power (3ph, Instantaneous)4" : powerlib_meascontrol/Measurements/Power (3ph, Instantaneous)
  Relational Operator1 : RelationalOperator  Operator=<=  OutDataTypeStr=boolean  RndMeth=Simplest
  Relational Operator2 : RelationalOperator  Operator=<=  OutDataTypeStr=boolean  RndMeth=Simplest
  Relational Operator3 : RelationalOperator  OutDataTypeStr=boolean  RndMeth=Nearest
  Relational Operator4 : RelationalOperator  Operator=<=  OutDataTypeStr=boolean  RndMeth=Nearest
  Relational Operator5 : RelationalOperator  OutDataTypeStr=boolean  RndMeth=Nearest
  Relay Operating Time : Display
  S-R Flip-Flop : simulink_extras/Flip Flops/S-R Flip-Flop  initial_condition=0
  Scope : Scope  NumInputPorts=8
  Scope1 : Scope  NumInputPorts=8
  Scope2 : Scope  NumInputPorts=8
  Subsystem : Subsystem
  Subsystem1 : Subsystem
  Subtract1 : Sum
  Subtract2 : Sum  Inputs=+-
  Subtract3 : Sum  Inputs=+-
  Subtract4 : Sum  Inputs=-+
  Subtract6 : Sum  Inputs=+-
  Switch1 : Switch  Criteria=u2 > Threshold  Threshold=pi
  Switch3 : Switch  Criteria=u2 > Threshold  Threshold=-pi
  Transport Delay : TransportDelay  DelayTime=0.01
  Meas : Outport
  SW Command : Outport  Port=2
  tag scope: Gen_outside_anglediff=global, Gen_outside_freqdiff=global
  wires:
  Abs1/1 -> Relational Operator2/1
  Abs/1 -> Relational Operator1/1
  Switch3/1 -> Switch1/2, Switch1/3, Subtract4/2
  Subtract4/1 -> Switch1/1
  Data Type Conversion/1 -> "   3"/1
  Relational Operator5/1 -> Scope/4, S-R Flip-Flop/1
  S-R Flip-Flop/1 -> Scope/5, Data Type Conversion/1
  Gain1/1 -> Mux4/12
  Gain/1 -> Mux4/11, Display/1
  2 kHz2/1 -> Gain1/1
  2 kHz1/1 -> Gain/1
  "   3"/1 -> Data Type Conversion2/1, Logical Operator1/2
  "Power (3ph, Instantaneous)4"/2 -> 2 kHz2/1
  Logical Operator7/1 -> Scope/8, Logical Operator2/2
  Status command/1 -> Logical Operator5/1, Mux4/13, Logical Operator2/1
  Logical Operator/1 -> Scope1/3, Scope2/3, Logical Operator7/3
  [Angle_diff] -> Relational Operator2/2
  [Freq_diff] -> Relational Operator1/2
  Subtract2/1 -> [Gen_outside_freqdiff], Scope1/1, Abs/1
  Relational Operator2/1 -> Logical Operator/3
  Relational Operator1/1 -> Logical Operator/2
  PLL (3ph)5/2 -> Subtract6/2
  Mux4/1 -> Meas/1
  PLL (3ph)4/2 -> Subtract6/1
  3Pto1P2/1(Va) -> Subsystem1/1(VaL), Subsystem/1(VaL), Mux4/2
  3Pto1P2/2(Vb) -> Mux4/3, Subsystem1/2(VbL), Subsystem/3(VbL)
  3Pto1P2/3(Vc) -> Subsystem1/3(VcL), Subsystem/5(VcL), Mux4/4
  3Pto1P1/1(Va) -> Mux4/5, Subsystem1/4(VaR), Subsystem/2(VaR)
  3Pto1P1/2(Vb) -> Subsystem1/5(VbR), Subsystem/4(VbR), Mux4/6
  3Pto1P1/3(Vc) -> Subsystem1/6(VcR), Subsystem/6(VcR), Mux4/7
  PLL (3ph)4/1 -> Mux4/8, Subtract2/1
  PLL (3ph)5/1 -> 2 kHz3/1, Mux4/9, Subtract2/2
  "Power (3ph, Instantaneous)4"/1 -> 2 kHz1/1
  Logical Operator2/1 -> Counter/1, Scope/1
  Constant1/1 -> Relational Operator5/2
  Counter/1 -> Scope/2, Counter1/1
  Counter1/1 -> Scope/3, Relational Operator5/1
  Subsystem/1(Vdiff) -> Logical Operator/1
  Subsystem1/1(VL) -> Scope2/1, Logical Operator7/1
  Subsystem1/2(VR) -> Scope2/2, Logical Operator7/2
  Voltage (Right)/1 -> Memory3/1, Scope1/6, Subtract3/2, PLL (3ph)5/1, 3Pto1P1/1(Vabc)
  Subtract6/1 -> Subtract1/2, Switch3/1, Switch3/2
  Constant7/1 -> Subtract1/1, Subtract4/1
  Subtract3/1 -> Scope1/7
  Subtract1/1 -> Switch3/3
  Voltage (Left)/1 -> Memory2/1, Subtract3/1, Scope1/5, "Power (3ph, Instantaneous)4"/1, PLL (3ph)4/1, 3Pto1P2/1(Vabc)
  Current/1 -> Fourier/1, Scope1/4, "Power (3ph, Instantaneous)4"/2, Memory1/1
  Irms1/1 -> ?
  Irms2/1 -> ?
  ? -> Relay Operating Time/1
  ? -> ?
  Memory2/1 -> Irms2/1
  Memory1/1 -> Detection/2(I), Irms1/1
  Detection/1(Direction) -> ?
  [RP_Y1_block_in] -> ?
  Memory3/1 -> Detection/1(V)
  ? -> Transport Delay/1, Logical Operator3/1
  Transport Delay/1 -> Logical Operator4/1
  Logical Operator3/1 -> Logical Operator6/1
  Logical Operator4/1 -> Logical Operator6/2
  Logical Operator6/1 -> Logical Operator8/1
  Fourier/1 -> Demux9/1
  Demux9/1 -> Mux4/15
  [Y1_OCRelay_F_DIR] -> ?
  [Y1_ManualReset] -> ?
  Logical Operator1/1 -> Data Type Conversion3/1
  Logical Operator8/1 -> Multiport Switch4/1
  Constant/1 -> Multiport Switch4/2
  Logical Operator9/1 -> Counter1/2
  Logical Operator5/1 -> Logical Operator9/2, S-R Flip-Flop/2
  Switch1/1 -> [Gen_outside_anglediff], Mux4/10, Scope1/2, Abs1/1
  Logical Operator11/1 -> Logical Operator10/1, Logical Operator1/1
  2 kHz3/1 -> Relational Operator4/1, Relational Operator3/1
  Constant2/1 -> Relational Operator3/2
  Relational Operator4/1 -> Logical Operator11/2
  Relational Operator3/1 -> Logical Operator11/1
  Constant3/1 -> Relational Operator4/2
  Logical Operator10/1 -> Logical Operator9/1
  Data Type Conversion1/1 -> Mux4/1
  Data Type Conversion2/1 -> Mux4/14
  Data Type Conversion3/1 -> Multiport Switch4/3, SW Command/1, Data Type Conversion1/1

== system PhaseII_opalrt_NoProtection/SM_System/Generator2/PI_Vd1 ==
  Error : Inport
  "Reset " : Inport  Port=2
  Add : Sum
  Add1 : Sum  Inputs=+-
  Constant25 : Constant
  D2 : Scope  NumInputPorts=2
  Delay : Delay  DelayLength=1
  Embedded MATLAB Function1 : MATLAB Function  TreatAsAtomicUnit=on
  Integrator1 : Integrator  ExternalReset=rising  InitialConditionSource=external  LimitOutput=on  UpperSaturationLimit=1  LowerSaturationLimit=-1
  K : Gain
  K1 : Gain
  K2 : Gain  Gain=Vabc_B
  K3 : Gain  Gain=-1
  Ki1 : Gain  Gain=0.1
  Kp1 : Gain  Gain=0
  Logical Operator : Logic  AllPortsSameDT=off  OutDataTypeStr=boolean
  PLL : powerlib_meascontrol/PLL/PLL  Fmin=58  Par_Init=[0, 60]  ParK=[180, 3200, 1]  TcD=1e-4  MaxRateChangeFreq=12  FilterCutOffFreq=25  Ts=0  AGC=on
  Relational Operator : RelationalOperator  Operator=<  OutDataTypeStr=boolean  ZeroCross=off  RndMeth=Nearest
  Relational Operator1 : RelationalOperator  Operator=>  OutDataTypeStr=boolean  ZeroCross=off  RndMeth=Nearest
  Out : Outport
  wires:
  Delay/1 -> Integrator1/3
  Add1/1 -> Delay/1
  ? -> Add1/1
  "Reset "/1 -> Integrator1/2
  Embedded MATLAB Function1/1(dout) -> Integrator1/1
  K1/1 -> Relational Operator1/1, Relational Operator/1, Out/1
  Logical Operator/1 -> Embedded MATLAB Function1/2(enable)
  Relational Operator/1 -> Logical Operator/1
  Relational Operator1/1 -> Logical Operator/2
  K3/1 -> Relational Operator1/2
  Add/1 -> K1/1
  K/1 -> Kp1/1, Ki1/1
  Ki1/1 -> Embedded MATLAB Function1/1(din)
  Kp1/1 -> Add/1, Add1/2
  Integrator1/1 -> Add/2, D2/1
  Constant25/1 -> K3/1, Relational Operator/2
  Error/1 -> D2/2, K/1

== system PhaseII_opalrt_NoProtection/SM_System/Generator2/PI_Vd10 ==
  Error : Inport
  "Reset " : Inport  Port=2
  Add : Sum
  Add1 : Sum  Inputs=+-
  Add2 : Sum  Inputs=+-
  Constant1 : Constant  Value=0.09
  Constant25 : Constant
  D2 : Scope  NumInputPorts=2
  Delay : Delay  DelayLength=1
  Embedded MATLAB Function1 : MATLAB Function  TreatAsAtomicUnit=on
  Integrator1 : Integrator  ExternalReset=rising  InitialConditionSource=external  LimitOutput=on  UpperSaturationLimit=1  LowerSaturationLimit=-1
  K : Gain
  K1 : Gain
  K3 : Gain  Gain=-1
  Ki1 : Gain  Gain=2
  Kp1 : Gain
  Logical Operator : Logic  AllPortsSameDT=off  OutDataTypeStr=boolean
  Relational Operator : RelationalOperator  Operator=<  OutDataTypeStr=boolean  ZeroCross=off  RndMeth=Nearest
  Relational Operator1 : RelationalOperator  Operator=>  OutDataTypeStr=boolean  ZeroCross=off  RndMeth=Nearest
  Out : Outport
  wires:
  Constant25/1 -> Relational Operator/2, K3/1
  Integrator1/1 -> D2/1, Add/2
  Kp1/1 -> Add1/2, Add/1
  Ki1/1 -> Embedded MATLAB Function1/1(din)
  K/1 -> Ki1/1, Kp1/1
  Add/1 -> K1/1
  K3/1 -> Relational Operator1/2
  Relational Operator1/1 -> Logical Operator/2
  Relational Operator/1 -> Logical Operator/1
  Logical Operator/1 -> Embedded MATLAB Function1/2(enable)
  K1/1 -> Out/1, Relational Operator/1, Relational Operator1/1
  Embedded MATLAB Function1/1(dout) -> Integrator1/1
  "Reset "/1 -> Integrator1/2
  [Gen_P] -> Add1/1
  Add1/1 -> Delay/1
  Delay/1 -> Integrator1/3
  Error/1 -> Add2/1
  Add2/1 -> K/1
  Constant1/1 -> Add2/2

== system PhaseII_opalrt_NoProtection/SM_System/Generator2/Subsystem2 ==
  Pe : Inport
  VdVqFB : Inport  Port=2
  2 kHz2 : dsparch4/Analog Filter Design  method=Butterworth  filttype=Lowpass  N=2  Wlo=2*pi*0.1  Whi=80  Rp=2  Rs=40
  Add1 : Sum
  Add2 : Sum
  Add3 : Sum  Inputs=++-+
  Constant1 : Constant
  Constant3 : Constant
  Constant4 : Constant  Value=2*pi
  Demux : Demux  Outputs=2
  Exciter : Subsystem
  Gain : Gain  Gain=2*pi*60
  Gain1 : Gain
  Gain2 : Gain
  Integrator : Integrator  InitialCondition=2*pi*60  ZeroCross=off
  Math Function : Math  Operator=square  SaturateOnIntegerOverflow=on
  Math Function1 : Math  Operator=square  SaturateOnIntegerOverflow=on
  Math Function2 : Math  Operator=mod  SaturateOnIntegerOverflow=on
  PSS : Subsystem
  Saturation : Saturate  UpperLimit=0.1  LowerLimit=-0.1  ZeroCross=off
  Sqrt : Sqrt  SaturateOnIntegerOverflow=on
  Voltage and Current Bus4 : Scope  NumInputPorts=3
  thermal_turbine_droop : Subsystem
  thermal_turbine_droop1 : Subsystem
  w : Outport
  Ef : Outport  Port=2
  rotor angle : Outport  Port=3
  tag scope: V2=global
  wires:
  thermal_turbine_droop/1(dww) -> Add1/1, PSS/1(dw), thermal_turbine_droop/1(dw)
  Integrator/1 -> Gain/1
  Gain/1 -> Math Function2/1
  Math Function2/1 -> rotor angle/1
  Constant4/1 -> Math Function2/2
  Constant3/1 -> Add1/2
  Add1/1 -> Integrator/1, Voltage and Current Bus4/1, w/1
  Add2/1 -> Sqrt/1
  Math Function1/1 -> Add2/2
  Math Function/1 -> Add2/1
  Sqrt/1 -> Exciter/1(Vt), [V2]
  Demux/1 -> Math Function/1
  Exciter/1(Ef) -> Ef/1
  Demux/2 -> Math Function1/1
  VdVqFB/1 -> Demux/1
  Pe/1 -> Voltage and Current Bus4/2, thermal_turbine_droop/2(pe)
  PSS/1(Vpss) -> Saturation/1
  Add3/1 -> Exciter/2(Vtr0)
  Constant1/1 -> Add3/1
  [Gen_V] -> Add3/2
  Saturation/1 -> Exciter/3(Vpss)
  [Q2] -> Gain1/1
  Gain1/1 -> Add3/3
  [Pe2] -> Gain2/1
  Gain2/1 -> 2 kHz2/1
  2 kHz2/1 -> Add3/4

== system PhaseII_opalrt_NoProtection/SM_System/Generator2/abc -> dq ==
  abc : Inport
  Theta : Inport  Port=2
  Demux : Demux  Outputs=3
  "abc -> dq" : Subsystem
  d : Outport
  q : Outport  Port=2
  0 : Outport  Port=3
  wires:
  "abc -> dq"/1(id) -> d/1
  abc/1 -> Demux/1
  "abc -> dq"/2(iq) -> q/1
  Demux/1 -> "abc -> dq"/1(a)
  Demux/2 -> "abc -> dq"/2(b)
  Demux/3 -> "abc -> dq"/3(c)
  Theta/1 -> "abc -> dq"/4(Theta)
  "abc -> dq"/3(i0) -> 0/1

== system PhaseII_opalrt_NoProtection/SM_System/Generator2/abc -> dq1 ==
  abc : Inport
  Theta : Inport  Port=2
  Demux : Demux  Outputs=3
  "abc -> dq" : Subsystem
  d : Outport
  q : Outport  Port=2
  0 : Outport  Port=3
  wires:
  "abc -> dq"/1(id) -> d/1
  abc/1 -> Demux/1
  "abc -> dq"/2(iq) -> q/1
  Demux/1 -> "abc -> dq"/1(a)
  Demux/2 -> "abc -> dq"/2(b)
  Demux/3 -> "abc -> dq"/3(c)
  Theta/1 -> "abc -> dq"/4(Theta)
  "abc -> dq"/3(i0) -> 0/1

== system PhaseII_opalrt_NoProtection/SM_System/Generator2/dq -> abc ==
  Theta : Inport
  dq : Inport  Port=2
  Demux : Demux  Outputs=2
  Mux : Mux  Inputs=3
  Transport Delay : TransportDelay  DelayTime=1e-6
  "dq -> abc" : Subsystem
  abc : Outport
  wires:
  "dq -> abc"/1(a) -> Mux/1
  "dq -> abc"/2(b) -> Mux/2
  "dq -> abc"/3(c) -> Mux/3
  Mux/1 -> Transport Delay/1
  Theta/1 -> "dq -> abc"/3(Theta)
  dq/1 -> Demux/1
  Demux/1 -> "dq -> abc"/1(d)
  Demux/2 -> "dq -> abc"/2(q)
  Transport Delay/1 -> abc/1

== system PhaseII_opalrt_NoProtection/SM_System/Generator2/electrical1 ==
  Efd : Inport
  IdIq : Inport  Port=2
  Add : Sum  Inputs=+-
  Add1 : Sum
  Add2 : Sum  Inputs=--
  Add3 : Sum  Inputs=++-
  Demux : Demux  Outputs=2
  Gain1 : Gain  Gain=xdp
  Gain2 : Gain  Gain=xq
  Gain3 : Gain  Gain=xqp
  Gain4 : Gain  Gain=1/Tq0p
  Gain5 : Gain  Gain=1/Td0p
  Gain6 : Gain  Gain=xd
  Integrator : Integrator  InitialCondition=-0.47  UpperSaturationLimit=10  LowerSaturationLimit=-10
  Integrator1 : Integrator  InitialCondition=1  UpperSaturationLimit=10  LowerSaturationLimit=-10
  Mux1 : Mux  Inputs=2
  Mux3 : Mux
  Saturation{,1..3} (4 alike) : Saturate  UpperLimit=2  LowerLimit=-2
  Te electrical torque : Fcn  Expr=u[1]*u[3]+u[2]*u[4]
  Voltage and Current Bus4 : Scope  NumInputPorts=3
  VdVqref : Outport
  Pe : Outport  Port=2
  wires:
  IdIq/1 -> Voltage and Current Bus4/3, Demux/1
  Mux1/1 -> VdVqref/1
  Mux3/1 -> Te electrical torque/1
  Gain4/1 -> Integrator/1
  Add2/1 -> Gain4/1
  Integrator/1 -> Saturation/1
  Gain3/1 -> Add/2
  Gain2/1 -> Add2/2
  Demux/2 -> Gain2/1, Gain3/1, Mux3/4
  Gain5/1 -> Integrator1/1
  Add3/1 -> Gain5/1
  Integrator1/1 -> Saturation1/1
  Efd/1 -> Add3/2
  Gain6/1 -> Add3/1
  Demux/1 -> Gain1/1, Gain6/1, Mux3/3
  Gain1/1 -> Add1/1
  Te electrical torque/1 -> Pe/1
  Add1/1 -> Saturation3/1, Add3/3
  Add/1 -> Saturation2/1, Add2/1
  Saturation/1 -> Add/1
  Saturation1/1 -> Add1/2
  Saturation2/1 -> Voltage and Current Bus4/1, Mux3/1, Mux1/1
  Saturation3/1 -> Voltage and Current Bus4/2, Mux3/2, Mux1/2

== system PhaseII_opalrt_NoProtection/SM_System/Generator2/line -> phase ==
  Vll : Inport
  Add1 : Sum  Inputs=+-
  Add2 : Sum  Inputs=+-
  Add3 : Sum  Inputs=+-
  Demux1 : Demux  Outputs=3
  Gain : Gain  Gain=1/3
  Mux : Mux  Inputs=3
  Vph : Outport
  wires:
  Demux1/1 -> Add1/1, Add2/2
  Demux1/3 -> Add1/2, Add3/1
  Demux1/2 -> Add2/1, Add3/2
  Add1/1 -> Mux/1
  Add2/1 -> Mux/2
  Add3/1 -> Mux/3
  Vll/1 -> Demux1/1
  Mux/1 -> Gain/1
  Gain/1 -> Vph/1

== system PhaseII_opalrt_NoProtection/SM_System/Generator2/line -> phase10 ==
  Vll : Inport
  Add1 : Sum  Inputs=+-
  Add2 : Sum  Inputs=+-
  Add3 : Sum  Inputs=+-
  Demux1 : Demux  Outputs=3
  Gain : Gain  Gain=1/3
  Mux : Mux  Inputs=3
  Vph : Outport
  wires:
  Demux1/1 -> Add1/1, Add2/2
  Demux1/3 -> Add1/2, Add3/1
  Demux1/2 -> Add2/1, Add3/2
  Add1/1 -> Mux/1
  Add2/1 -> Mux/2
  Add3/1 -> Mux/3
  Vll/1 -> Demux1/1
  Mux/1 -> Gain/1
  Gain/1 -> Vph/1
